simulink model "AM_V2"  (R2022a)
settings: Solver=VariableStepAuto  StartTime=0.0  StopTime=10.0  RelTol=1e-3
settings Model: Creator=Yogesh  LastModifiedBy=Yogesh

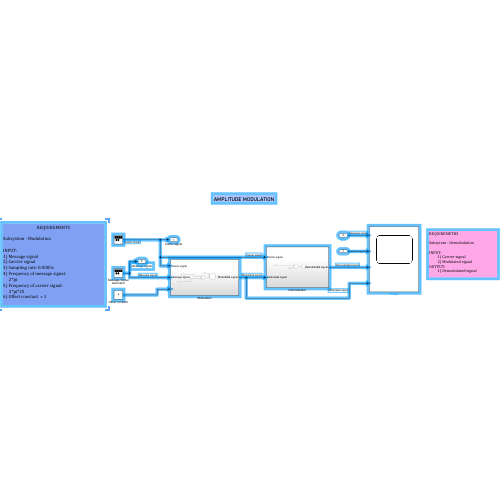
[thumbnail: Simulink's stored preview of the top-level diagram]
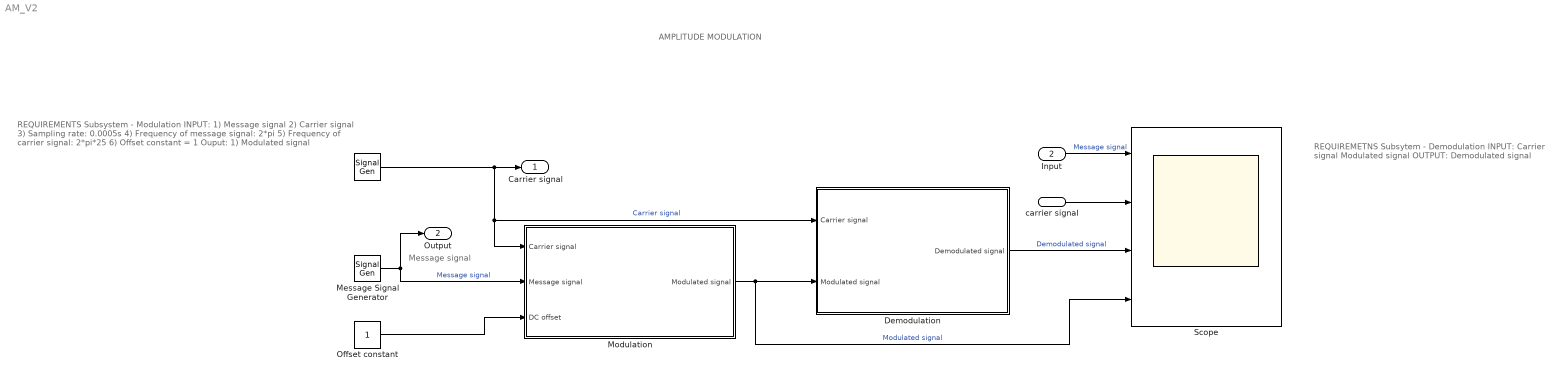
== system AM_V2 ==
  note: REQUIREMETNS
      |
      | Subsytem - Demodulation
      |
      | INPUT:
      | Carrier signal
      | Modulated signal
      | OUTPUT:
      | Demodulated signal
  note: REQUIREMENTS
      |
      | Subsystem - Modulation
      |
      | INPUT:
      | 1) Message signal
      | 2) Carrier signal
      | 3) Sampling rate: 0.0005s
      | 4) Frequency of message signal:
      | 2*pi
      | 5) Frequency of carrier signal:
      | 2*pi*25
      | 6) Offset constant = 1
      |
      | Ouput:
      | 1) Modulated signal
  note: AMPLITUDE MODULATION
  note: Message signal
  carrier signal : Inport
  Input : Inport  Port=2
  " " : SignalGenerator  Frequency=2*pi*25  Units=rad/sec
  Demodulation : Subsystem
  Message Signal Generator : SignalGenerator  Frequency=2*pi  Units=rad/sec
  Modulation : Subsystem
  Offset constant : Constant
  Scope : Scope  NumInputPorts=4
  Carrier signal : Outport
  Output : Outport  Port=2
  wires:
  " "/1 -> Carrier signal/1, Demodulation/1(Carrier signal), Modulation/1(Carrier signal)  "Carrier signal"
  Message Signal Generator/1 -> Output/1, Modulation/2(Message signal)  "Message signal"
  Modulation/1(Modulated signal) -> Demodulation/2(Modulated signal), Scope/4  "Modulated signal"
  Offset constant/1 -> Modulation/3(DC offset)
  carrier signal/1 -> Scope/2
  Input/1 -> Scope/1  "Message signal"
  Demodulation/1(Demodulated signal) -> Scope/3  "Demodulated signal"

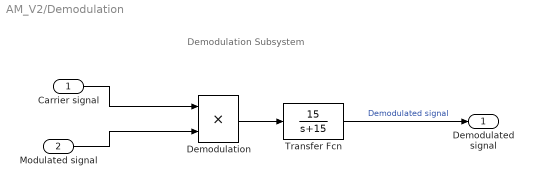
== system AM_V2/Demodulation ==
  note: Demodulation Subsystem
  Carrier signal : Inport
  Modulated signal : Inport  Port=2
  Demodulation : Product
  Transfer Fcn : TransferFcn  Numerator=[15]  Denominator=[1 15]
  Demodulated signal : Outport
  wires:
  Modulated signal/1 -> Demodulation/2
  Demodulation/1 -> Transfer Fcn/1
  Transfer Fcn/1 -> Demodulated signal/1  "Demodulated signal"
  Carrier signal/1 -> Demodulation/1

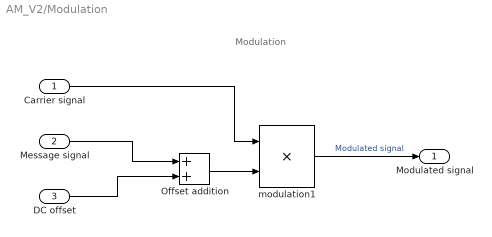
== system AM_V2/Modulation ==
  note: Modulation
  Carrier signal : Inport
  Message signal : Inport  Port=2
  DC offset : Inport  Port=3
  Offset addition : Sum
  modulation1 : Product
  Modulated signal : Outport
  wires:
  modulation1/1 -> Modulated signal/1  "Modulated signal"
  Offset addition/1 -> modulation1/2
  Carrier signal/1 -> modulation1/1
  Message signal/1 -> Offset addition/1
  DC offset/1 -> Offset addition/2
